simulink model "satellite1"  (Simulink 7.5)
settings: Solver=ode45  StartTime=0.0  StopTime=10.0  RelTol=1e-3
libraries: commseqgen2 x2, commsynccomp2 x2, commnoisgen2 x1, dspsrcs4 x1
settings Model: Creator=sisa  LastModifiedBy=SISA
settings SimEventsCC: propDiagAttribOutput=1  propDiagFcnCallOutput=1  propDiagStatOutput=0

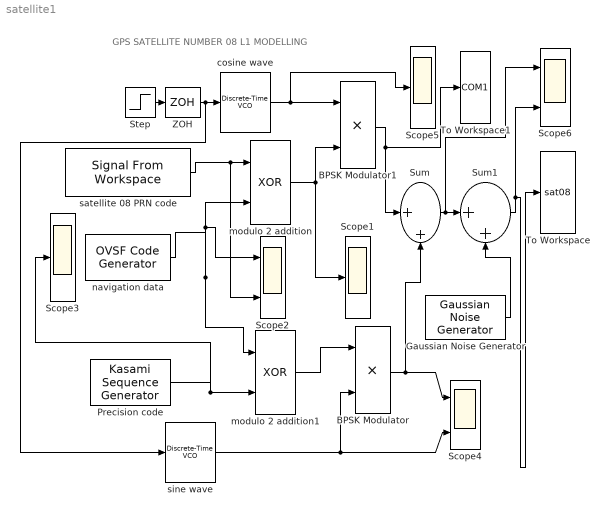
== system satellite1 ==
  note: GPS SATELLITE NUMBER 08 L1 MODELLING
  BPSK Modulator : Product  OutDataType=fixdt(1, 16)  OutScaling=2^0  RndMeth=Zero
  BPSK Modulator1 : Product  OutDataType=fixdt(1, 16)  OutScaling=2^0  RndMeth=Zero
  Gaussian Noise Generator : commnoisgen2/Gaussian Noise Generator  SystemSampleTime=-1  m=0  d=1  s=41  Ts=1  frameBased=off  sampPerFrame=1  orient=off  outDataType=double
  Precision code : commseqgen2/Kasami Sequence Generator  genPoly=[1 0 0 0 0 1 1]  iniState=[0 0 0 0 0 1]  codeIdx=0  shift=0  ts=1  frameBased=off  sampPerFrame=1  reset=off  outDataType=double
  Scope1 : Scope
  Scope2 : Scope  NumInputPorts=2
      settings: YMin=-5~-5  YMax=5~5
  Scope3 : Scope
      settings: SaveName=ScopeData2
  Scope4 : Scope  NumInputPorts=2
      settings: YMin=-5~-5  YMax=5~5  SaveName=ScopeData3
  Scope5 : Scope
      settings: SaveName=ScopeData4
  Scope6 : Scope  NumInputPorts=2
      settings: YMin=-5~-5  YMax=5~5  SaveName=ScopeData5
  Step : Step  After=2  SampleTime=0
  Sum : Sum  Inputs=|++  OutDataType=fixdt(1, 16)  OutScaling=2^0
  Sum1 : Sum  Inputs=|++  OutDataType=fixdt(1, 16)  OutScaling=2^0
  To Workspace : ToWorkspace  VariableName=sat08  SampleTime=-1  SaveFormat=Array
      settings: MaxDataPoints=1023000
  To Workspace1 : ToWorkspace  VariableName=COM1  SampleTime=-1  SaveFormat=Array
      settings: MaxDataPoints=1023000
  ZOH : ZeroOrderHold
  cosine wave : commsynccomp2/Discrete-Time VCO  SystemSampleTime=-1  Ac=3  Fc=7000000  Kc=1  Ph=0  ts=0.01
  modulo 2 addition : Logic  Operator=XOR  IconShape=distinctive  AllPortsSameDT=off  OutDataTypeMode=boolean  LogicDataType=fixdt(0, 8)  OutDataTypeStr=boolean
  modulo 2 addition1 : Logic  Operator=XOR  IconShape=distinctive  AllPortsSameDT=off  OutDataTypeMode=boolean  LogicDataType=fixdt(0, 8)  OutDataTypeStr=boolean
  navigation data : commseqgen2/OVSF Code Generator  SystemSampleTime=-1  spreadFact=1024  index=1023  ts=1  frameBased=off  sampPerFrame=1  outDataType=double
  satellite 08 PRN code : dspsrcs4/Signal From Workspace  SystemSampleTime=-1  X=PN08  Ts=1  nsamps=1  OutputAfterFinalValue=Setting to zero  ignoreOrWarnInputAndFrameLengths=off
  sine wave : commsynccomp2/Discrete-Time VCO  SystemSampleTime=-1  Ac=3  Fc=7000000  Kc=1  Ph=-pi/2  ts=0.01
  wires:
  satellite 08 PRN code/1 -> modulo 2 addition/1, Scope2/2
  BPSK Modulator1/1 -> Sum/1, To Workspace1/1
  modulo 2 addition/1 -> BPSK Modulator1/2, Scope1/1
  Step/1 -> ZOH/1
  ZOH/1 -> cosine wave/1, sine wave/1
  cosine wave/1 -> BPSK Modulator1/1, Scope5/1
  navigation data/1 -> modulo 2 addition1/1, modulo 2 addition/2, Scope2/1
  modulo 2 addition1/1 -> BPSK Modulator/1
  sine wave/1 -> BPSK Modulator/2, Scope4/2
  Precision code/1 -> modulo 2 addition1/2, Scope3/1
  BPSK Modulator/1 -> Scope4/1, Sum/2
  Sum/1 -> Sum1/1, Scope6/1
  Gaussian Noise Generator/1 -> Sum1/2
  Sum1/1 -> Scope6/2, To Workspace/1
